simulink model "induct_closedloop_sim"  (Simulink 10.2)
settings: Solver=ode1  StartTime=0.0  StopTime=4  FixedStep=.000001  RelTol=1e-6  AbsTol=1e-6  EnableMultiTasking=on
values from neighbouring files (symbols this model uses):
  beta = M/(sigma*Lr*Ls)    (= 197.93605143)    [data_induct_closedloop.m]    (also in data_induct_closedloop_180turn.m)
  c1 = 3*wmax/(t1*t1)    (= 1066.66666667)    [data_induct_closedloop.m]    (also in data_induct_closedloop_180turn.m = 360000)
  c2 = -2*wmax/(t1*t1*t1)    (= -474.074074074)    [data_induct_closedloop.m]    (also in data_induct_closedloop_180turn.m = -9600000)
  d1 = 3*wmax/((t3-t2)*(t3-t2))    (= 1066.66666667)    [data_induct_closedloop.m]    (also in data_induct_closedloop_180turn.m = 360000)
  d2 = -2*wmax/((t3-t2)*(t3-t2)*(t3-t2))    (= -474.074074074)    [data_induct_closedloop.m]    (also in data_induct_closedloop_180turn.m = -9600000)
  eta = Rr/Lr    (= 278.571428571)    [data_induct_closedloop.m]    (also in data_induct_closedloop_180turn.m)
  eta2 = Rr/Lr    (= 278.571428571)    [data_induct_closedloop.m]    (also in data_induct_closedloop_180turn.m)
  f = 0    [data_induct_closedloop.m]    (also in data_induct_closedloop_180turn.m)
  gamma = M*M*Rr/(sigma*Lr*Lr*Ls) + Rs/(sigma*Ls)    (= 1047.76929212)    [data_induct_closedloop.m]    (also in data_induct_closedloop_180turn.m)
  id0 = 5.5/sqrt(2)    [data_induct_closedloop.m]    (also in data_induct_closedloop_180turn.m)
  Imax = 6    [data_induct_closedloop.m]    (also in data_induct_closedloop_180turn.m)
  J = 0.00011    [data_induct_closedloop.m]    (also in data_induct_closedloop_180turn.m)
  k0 = p0*p1*p2    (= 1000)    [data_induct_closedloop.m]    (also in data_induct_closedloop_180turn.m = 1000000)
  k1 = p0*p1 + p0*p2 + p1*p2    (= 300)    [data_induct_closedloop.m]    (also in data_induct_closedloop_180turn.m = 30000)
  k2 = p0+p1+p2    (= 30)    [data_induct_closedloop.m]    (also in data_induct_closedloop_180turn.m = 300)
  KI = 100*100    (= 10000)    [data_induct_closedloop.m]    (also in data_induct_closedloop_180turn.m = 1000000)
  KIf = 420000    [data_induct_closedloop.m]    (also in data_induct_closedloop_180turn.m)
  Kp = 100+100    (= 200)    [data_induct_closedloop.m]    (also in data_induct_closedloop_180turn.m = 2000)
  KPf = 10000    [data_induct_closedloop.m]    (also in data_induct_closedloop_180turn.m)
  KT2 = np*M2/Lr2    (= 2.50714285714)    [data_induct_closedloop.m]    (also in data_induct_closedloop_180turn.m)
  Lr = 0.014    [data_induct_closedloop.m]    (also in data_induct_closedloop_180turn.m)
  Ls = 0.014    [data_induct_closedloop.m]    (also in data_induct_closedloop_180turn.m)
  M = 0.0117    [data_induct_closedloop.m]    (also in data_induct_closedloop_180turn.m)
  M2 = M    (= 0.0117)    [data_induct_closedloop.m]    (also in data_induct_closedloop_180turn.m)
  mu = np*M/(J*Lr)    (= 22792.2077922)    [data_induct_closedloop.m]    (also in data_induct_closedloop_180turn.m)
  np = 3    [data_induct_closedloop.m]    (also in data_induct_closedloop_180turn.m)
  sigma = 1 - M*M/(Lr*Ls)    (= 0.301581632653)    [data_induct_closedloop.m]    (also in data_induct_closedloop_180turn.m)
  t3 = t2 + t1    (= 3.1)    [data_induct_closedloop.m]    (also in data_induct_closedloop_180turn.m = 0.0668879020479)
  tau_L = 0    [data_induct_closedloop.m]    (also in data_induct_closedloop_180turn.m)
  tdd = 0.01    [data_induct_closedloop.m]    (also in data_induct_closedloop_180turn.m)
  Vmax = V    (= 60)    [data_induct_closedloop.m]    (also in data_induct_closedloop_180turn.m)
  wbase = 250    [data_induct_closedloop.m]    (also in data_induct_closedloop_180turn.m)
undefined symbols (not defined in the file or in its folder): integrator_sat
libraries: simulink x2
settings Model: Creator=johnchiasson  LastModifiedBy=johnchiasson  ExtModeTrigMode=oneshot  ExtModeArmWhenConnect=off
settings DataIOCC: SignalLoggingName=sigsOut
settings OptimizationCC: BlockReduction=off  BooleanDataType=off  LifeSpan=auto
settings DebuggingCC: SaveWithParameterizedLinksMsg=none  SignalResolutionControl=TryResolveAllWithWarning  MultiTaskDSMMsg=warning  MultiTaskCondExecSysMsg=none  FcnCallInpInsideContextMsg=error  SFUnexpectedBacktrackingDiag=error  SFNoUnconditionalDefaultTransitionDiag=error  SFExecutionAtInitializationDiag=warning  ArithmeticOperatorsInVariantConditions=error
settings HardwareCC: TargetUnknown=on
settings SFSimCC: SimUseLocalCustomCode=on  CustomCodeUndefinedFunction=FilterOut
settings RTWCC: RTWUseLocalCustomCode=on
settings CodeAppCC: StateflowObjectComments=off
settings GRTTargetCC: TargetLangStandard=C99 (ISO)
settings ConfigComp: CovExternalEMLEnable=on

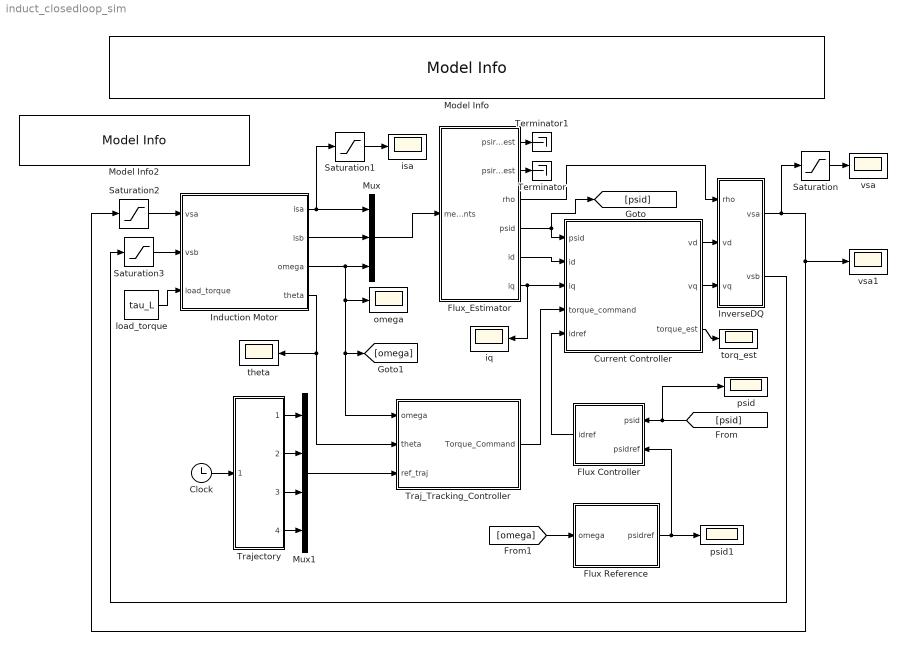
== system induct_closedloop_sim ==
  Clock : Clock
  Current Controller : Subsystem
  Flux Controller : Subsystem
  Flux Reference : Subsystem
  Flux_Estimator : Subsystem
  Induction Motor : Subsystem
  InverseDQ : Subsystem
  Model Info : simulink/Model-Wide Utilities/Model Info  Frame=on  DisplayStringWithTags=Simulation of an Input-Output Linearization Controller High Speed Run  HorizontalTextAlignment=Center  LeftAlignmentValue=0.5
  Model Info2 : simulink/Model-Wide Utilities/Model Info  Frame=on  DisplayStringWithTags="To initialize the simulation run  data_induct_closedloop.m"  HorizontalTextAlignment=Center  LeftAlignmentValue=0.5
  Mux : Mux  Inputs=3
  Mux1 : Mux
  Saturation : Saturate  UpperLimit=Vmax  LowerLimit=-Vmax
  Saturation1 : Saturate  UpperLimit=Imax  LowerLimit=-Imax
  Saturation2 : Saturate  UpperLimit=Vmax  LowerLimit=-Vmax
  Saturation3 : Saturate  UpperLimit=Vmax  LowerLimit=-Vmax
  Terminator : Terminator
  Terminator1 : Terminator
  Traj_Tracking_Controller : Subsystem
  Trajectory : Subsystem
  iq : Scope
  isa : Scope
  load_torque : Constant  Value=tau_L
  omega : Scope
  psid : Scope
  psid1 : Scope
  theta : Scope
  torq_est : Scope
  vsa : Scope
  vsa1 : Scope
  wires:
  load_torque/1 -> Induction Motor/3(load_torque)
  Mux/1 -> Flux_Estimator/1(measurements)
  Induction Motor/3(omega) -> Mux/3, Traj_Tracking_Controller/1(omega), [omega], omega/1
  Induction Motor/2(isb) -> Mux/2
  Induction Motor/1(isa) -> Mux/1, Saturation1/1
  Flux_Estimator/5(id) -> Current Controller/2(id)
  Flux_Estimator/6(iq) -> Current Controller/3(iq), iq/1
  Flux_Estimator/4(psid) -> Current Controller/1(psid), [psid]
  Current Controller/3(torque_est) -> torq_est/1
  Flux_Estimator/3(rho) -> InverseDQ/1(rho)
  Current Controller/1(vd) -> InverseDQ/2(vd)
  Current Controller/2(vq) -> InverseDQ/3(vq)
  Clock/1 -> Trajectory/1(time)
  Mux1/1 -> Traj_Tracking_Controller/3(ref_traj)
  Trajectory/4(jerk_ref) -> Mux1/4
  Trajectory/1(theta_ref) -> Mux1/1
  Trajectory/2(omega_ref) -> Mux1/2
  Trajectory/3(alpha_ref) -> Mux1/3
  InverseDQ/1(vsa) -> Saturation/1, Saturation2/1, vsa1/1
  InverseDQ/2(vsb) -> Saturation3/1
  Induction Motor/4(theta) -> Traj_Tracking_Controller/2(theta), theta/1
  Traj_Tracking_Controller/1(Torque_Command) -> Current Controller/4(torque_command)
  [psid] -> Flux Controller/1(psid), psid/1
  Flux Controller/1(idref) -> Current Controller/5(idref)
  Flux_Estimator/1(psira_est) -> Terminator1/1
  Flux_Estimator/2(psirb_est) -> Terminator/1
  Flux Reference/1(psidref) -> psid1/1, Flux Controller/2(psidref)
  [omega] -> Flux Reference/1(omega)
  Saturation/1 -> vsa/1
  Saturation1/1 -> isa/1
  Saturation2/1 -> Induction Motor/1(vsa)
  Saturation3/1 -> Induction Motor/2(vsb)

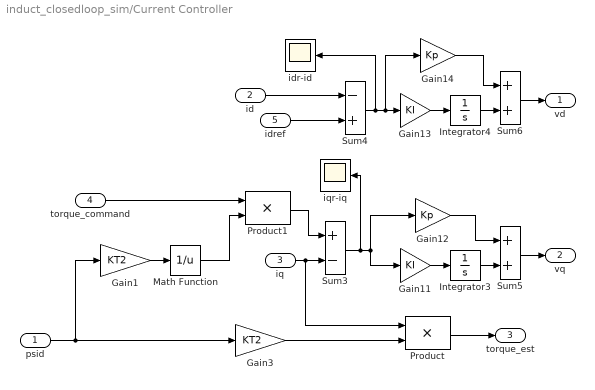
== system induct_closedloop_sim/Current Controller ==
  psid : Inport
  id : Inport  Port=2
  iq : Inport  Port=3
  torque_command : Inport  Port=4
  idref : Inport  Port=5
  Gain1 : Gain  Gain=KT2  SaturateOnIntegerOverflow=on  OutDataTypeStr=Inherit: Same as input  ParamDataTypeStr=Inherit: Same as input
  Gain11 : Gain  Gain=KI  SaturateOnIntegerOverflow=on  OutDataTypeStr=Inherit: Same as input  ParamDataTypeStr=Inherit: Same as input
  Gain12 : Gain  Gain=Kp  SaturateOnIntegerOverflow=on  OutDataTypeStr=Inherit: Same as input  ParamDataTypeStr=Inherit: Same as input
  Gain13 : Gain  Gain=KI  SaturateOnIntegerOverflow=on  OutDataTypeStr=Inherit: Same as input  ParamDataTypeStr=Inherit: Same as input
  Gain14 : Gain  Gain=Kp  SaturateOnIntegerOverflow=on  OutDataTypeStr=Inherit: Same as input  ParamDataTypeStr=Inherit: Same as input
  Gain3 : Gain  Gain=KT2  SaturateOnIntegerOverflow=on  OutDataTypeStr=Inherit: Same as input  ParamDataTypeStr=Inherit: Same as input
  Integrator3 : Integrator
  Integrator4 : Integrator
  Math Function : Math  Operator=reciprocal  SignedPower=on  SaturateOnIntegerOverflow=on
  Product : Product  InputSameDT=on  SaturateOnIntegerOverflow=on  OutDataTypeStr=Inherit: Same as first input
  Product1 : Product  InputSameDT=on  SaturateOnIntegerOverflow=on  OutDataTypeStr=Inherit: Same as first input
  Sum3 : Sum  Inputs=+-  InputSameDT=on  SaturateOnIntegerOverflow=on  OutDataTypeStr=Inherit: Same as first input
  Sum4 : Sum  Inputs=-+  InputSameDT=on  SaturateOnIntegerOverflow=on  OutDataTypeStr=Inherit: Same as first input
  Sum5 : Sum  InputSameDT=on  SaturateOnIntegerOverflow=on  OutDataTypeStr=Inherit: Same as first input
  Sum6 : Sum  InputSameDT=on  SaturateOnIntegerOverflow=on  OutDataTypeStr=Inherit: Same as first input
  idr-id : Scope
  iqr-iq : Scope
  vd : Outport
  vq : Outport  Port=2
  torque_est : Outport  Port=3
  wires:
  Sum4/1 -> idr-id/1, Gain13/1, Gain14/1
  Sum3/1 -> iqr-iq/1, Gain11/1, Gain12/1
  Gain12/1 -> Sum5/1
  Integrator3/1 -> Sum5/2
  Gain11/1 -> Integrator3/1
  Gain14/1 -> Sum6/1
  Gain13/1 -> Integrator4/1
  Sum6/1 -> vd/1
  id/1 -> Sum4/1
  idref/1 -> Sum4/2
  Product1/1 -> Sum3/1
  Sum5/1 -> vq/1
  iq/1 -> Sum3/2, Product/1
  Integrator4/1 -> Sum6/2
  Gain3/1 -> Product/2
  Product/1 -> torque_est/1
  psid/1 -> Gain3/1, Gain1/1
  torque_command/1 -> Product1/1
  Math Function/1 -> Product1/2
  Gain1/1 -> Math Function/1

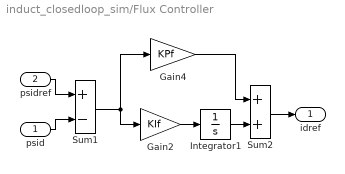
== system induct_closedloop_sim/Flux Controller ==
  psid : Inport
  psidref : Inport  Port=2
  Gain2 : Gain  Gain=KIf  SaturateOnIntegerOverflow=on  OutDataTypeStr=Inherit: Same as input  ParamDataTypeStr=Inherit: Same as input
  Gain4 : Gain  Gain=KPf  SaturateOnIntegerOverflow=on  OutDataTypeStr=Inherit: Same as input  ParamDataTypeStr=Inherit: Same as input
  Integrator1 : Integrator
  Sum1 : Sum  Inputs=+-  InputSameDT=on  SaturateOnIntegerOverflow=on  OutDataTypeStr=Inherit: Same as first input
  Sum2 : Sum  InputSameDT=on  SaturateOnIntegerOverflow=on  OutDataTypeStr=Inherit: Same as first input
  idref : Outport
  wires:
  Sum1/1 -> Gain2/1, Gain4/1
  Gain4/1 -> Sum2/1
  Integrator1/1 -> Sum2/2
  Gain2/1 -> Integrator1/1
  Sum2/1 -> idref/1
  psidref/1 -> Sum1/1
  psid/1 -> Sum1/2

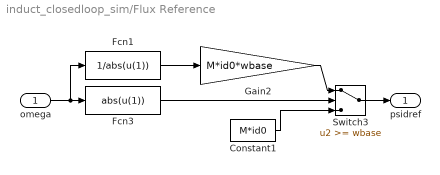
== system induct_closedloop_sim/Flux Reference ==
  omega : Inport
  Constant1 : Constant  Value=M*id0
  Fcn1 : Fcn  Expr=1/abs(u(1))
  Fcn3 : Fcn  Expr=abs(u(1))
  Gain2 : Gain  Gain=M*id0*wbase  SaturateOnIntegerOverflow=on  OutDataTypeStr=Inherit: Same as input  ParamDataTypeStr=Inherit: Same as input
  Switch3 : Switch  Threshold=wbase  SaturateOnIntegerOverflow=on  InputSameDT=on
  psidref : Outport
  wires:
  Gain2/1 -> Switch3/1
  Fcn3/1 -> Switch3/2
  omega/1 -> Fcn1/1, Fcn3/1
  Fcn1/1 -> Gain2/1
  Constant1/1 -> Switch3/3
  Switch3/1 -> psidref/1

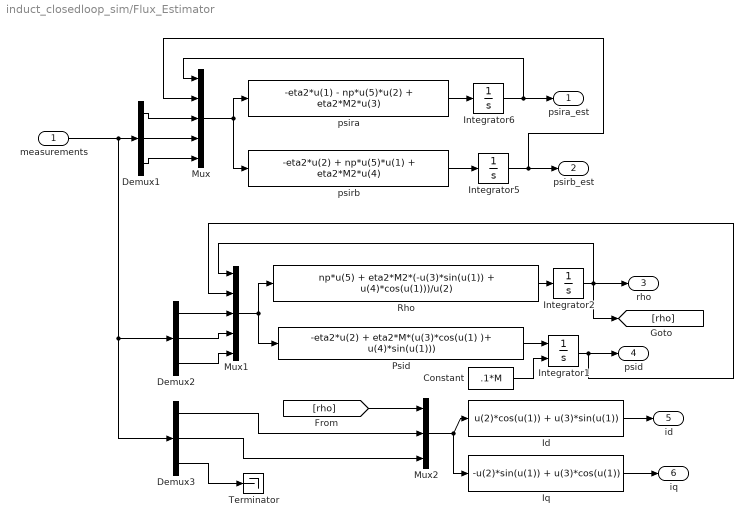
== system induct_closedloop_sim/Flux_Estimator ==
  measurements : Inport
  Constant : Constant  Value=.1*M
  Demux1 : Demux  Outputs=3
      settings: DisplayOption=none
  Demux2 : Demux  Outputs=3
      settings: DisplayOption=none
  Demux3 : Demux  Outputs=3
      settings: DisplayOption=none
  Id : Fcn  Expr=u(2)*cos(u(1)) + u(3)*sin(u(1))
  Integrator1 : Integrator  InitialConditionSource=external  UpperSaturationLimit=integrator_sat  LowerSaturationLimit=-integrator_sat
  Integrator2 : Integrator  UpperSaturationLimit=integrator_sat  LowerSaturationLimit=-integrator_sat
  Integrator5 : Integrator  UpperSaturationLimit=integrator_sat  LowerSaturationLimit=-integrator_sat
  Integrator6 : Integrator  UpperSaturationLimit=integrator_sat  LowerSaturationLimit=-integrator_sat
  Iq : Fcn  Expr=-u(2)*sin(u(1)) + u(3)*cos(u(1))
  Mux : Mux  Inputs=5
  Mux1 : Mux  Inputs=5
  Mux2 : Mux  Inputs=3
  Psid : Fcn  Expr=-eta2*u(2) + eta2*M*(u(3)*cos(u(1) )+ u(4)*sin(u(1)))
  Rho : Fcn  Expr=np*u(5) + eta2*M2*(-u(3)*sin(u(1)) + u(4)*cos(u(1)))/u(2)
  Terminator : Terminator
  psira : Fcn  Expr=-eta2*u(1) - np*u(5)*u(2) + eta2*M2*u(3)
  psirb : Fcn  Expr=-eta2*u(2) + np*u(5)*u(1) + eta2*M2*u(4)
  psira_est : Outport
  psirb_est : Outport  Port=2
  rho : Outport  Port=3
  psid : Outport  Port=4
  id : Outport  Port=5
  iq : Outport  Port=6
  wires:
  psirb/1 -> Integrator5/1
  psira/1 -> Integrator6/1
  Integrator6/1 -> psira_est/1, Mux/1
  Integrator5/1 -> psirb_est/1, Mux/2
  Mux/1 -> psira/1, psirb/1
  Psid/1 -> Integrator1/1
  Rho/1 -> Integrator2/1
  Integrator2/1 -> rho/1, Mux1/1, [rho]
  Integrator1/1 -> psid/1, Mux1/2
  Mux1/1 -> Rho/1, Psid/1
  Id/1 -> id/1
  Iq/1 -> iq/1
  Demux3/1 -> Mux2/2
  Demux3/3 -> Terminator/1
  Demux3/2 -> Mux2/3
  [rho] -> Mux2/1
  Mux2/1 -> Id/1, Iq/1
  Constant/1 -> Integrator1/2
  measurements/1 -> Demux1/1, Demux2/1, Demux3/1
  Demux1/1 -> Mux/3
  Demux1/2 -> Mux/4
  Demux1/3 -> Mux/5
  Demux2/1 -> Mux1/3
  Demux2/2 -> Mux1/4
  Demux2/3 -> Mux1/5

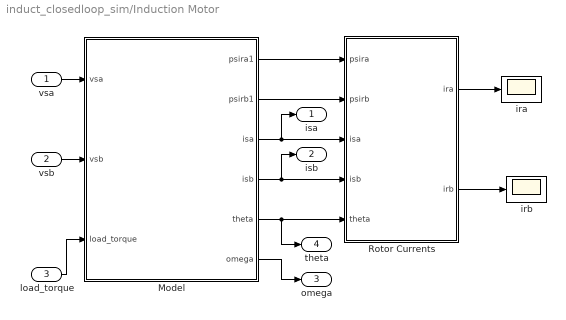
== system induct_closedloop_sim/Induction Motor ==
  vsa : Inport
  vsb : Inport  Port=2
  load_torque : Inport  Port=3
  Model : Subsystem
  Rotor Currents : Subsystem
  ira : Scope
  irb : Scope
  isa : Outport
  isb : Outport  Port=2
  omega : Outport  Port=3
  theta : Outport  Port=4
  wires:
  Model/1(psira1) -> Rotor Currents/1(psira)
  Model/2(psirb1) -> Rotor Currents/2(psirb)
  Model/3(isa) -> Rotor Currents/3(isa), isa/1
  Model/4(isb) -> Rotor Currents/4(isb), isb/1
  Model/6(omega) -> omega/1
  vsa/1 -> Model/1(vsa)
  vsb/1 -> Model/2(vsb)
  load_torque/1 -> Model/3(load_torque)
  Model/5(theta) -> theta/1, Rotor Currents/5(theta)
  Rotor Currents/1(ira) -> ira/1
  Rotor Currents/2(irb) -> irb/1

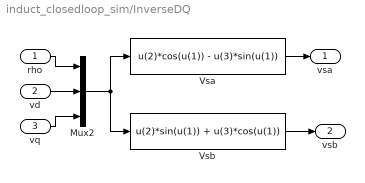
== system induct_closedloop_sim/InverseDQ ==
  rho : Inport
  vd : Inport  Port=2
  vq : Inport  Port=3
  Mux2 : Mux  Inputs=3
  Vsa : Fcn  Expr=u(2)*cos(u(1)) - u(3)*sin(u(1))
  Vsb : Fcn  Expr=u(2)*sin(u(1)) + u(3)*cos(u(1))
  vsa : Outport
  vsb : Outport  Port=2
  wires:
  Vsa/1 -> vsa/1
  Vsb/1 -> vsb/1
  Mux2/1 -> Vsa/1, Vsb/1
  rho/1 -> Mux2/1
  vd/1 -> Mux2/2
  vq/1 -> Mux2/3

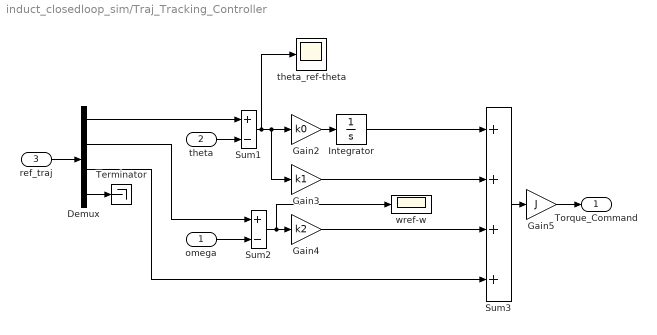
== system induct_closedloop_sim/Traj_Tracking_Controller ==
  omega : Inport
  theta : Inport  Port=2
  ref_traj : Inport  Port=3
  Demux : Demux
      settings: DisplayOption=none
  Gain2 : Gain  Gain=k0  SaturateOnIntegerOverflow=on  OutDataTypeStr=Inherit: Same as input  ParamDataTypeStr=Inherit: Same as input
  Gain3 : Gain  Gain=k1  SaturateOnIntegerOverflow=on  OutDataTypeStr=Inherit: Same as input  ParamDataTypeStr=Inherit: Same as input
  Gain4 : Gain  Gain=k2  SaturateOnIntegerOverflow=on  OutDataTypeStr=Inherit: Same as input  ParamDataTypeStr=Inherit: Same as input
  Gain5 : Gain  Gain=J  SaturateOnIntegerOverflow=on  OutDataTypeStr=Inherit: Same as input  ParamDataTypeStr=Inherit: Same as input
  Integrator : Integrator
  Sum1 : Sum  Inputs=+-  InputSameDT=on  SaturateOnIntegerOverflow=on  OutDataTypeStr=Inherit: Same as first input
  Sum2 : Sum  Inputs=+-  InputSameDT=on  SaturateOnIntegerOverflow=on  OutDataTypeStr=Inherit: Same as first input
  Sum3 : Sum  Inputs=++++  InputSameDT=on  SaturateOnIntegerOverflow=on  OutDataTypeStr=Inherit: Same as first input
  Terminator : Terminator
  theta_ref-theta : Scope
  wref-w : Scope
  Torque_Command : Outport
  wires:
  Demux/1 -> Sum1/1
  Gain2/1 -> Integrator/1
  Integrator/1 -> Sum3/1
  theta/1 -> Sum1/2
  ref_traj/1 -> Demux/1
  Demux/4 -> Terminator/1
  Demux/2 -> Sum2/1
  Gain4/1 -> Sum3/3
  Sum3/1 -> Gain5/1
  Sum1/1 -> Gain2/1, Gain3/1, theta_ref-theta/1
  Sum2/1 -> Gain4/1, wref-w/1
  Gain3/1 -> Sum3/2
  Gain5/1 -> Torque_Command/1
  omega/1 -> Sum2/2
  Demux/3 -> Sum3/4

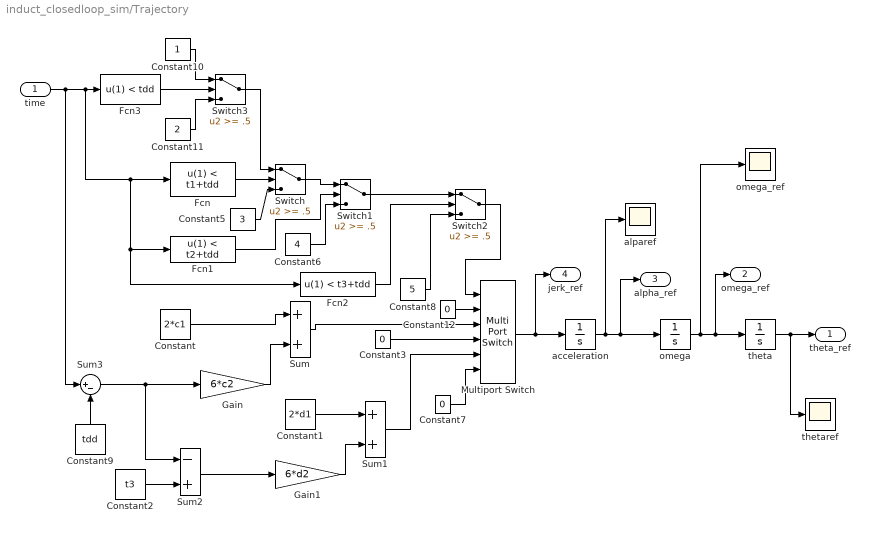
== system induct_closedloop_sim/Trajectory ==
  time : Inport
  Constant : Constant  Value=2*c1
  Constant1 : Constant  Value=2*d1
  Constant10 : Constant
  Constant11 : Constant  Value=2
  Constant12 : Constant  Value=0
  Constant2 : Constant  Value=t3
  Constant3 : Constant  Value=0
  Constant5 : Constant  Value=3
  Constant6 : Constant  Value=4
  Constant7 : Constant  Value=0
  Constant8 : Constant  Value=5
  Constant9 : Constant  Value=tdd
  Fcn : Fcn  Expr=u(1) < t1+tdd
  Fcn1 : Fcn  Expr=u(1) < t2+tdd
  Fcn2 : Fcn  Expr=u(1) < t3+tdd
  Fcn3 : Fcn  Expr=u(1) < tdd
  Gain : Gain  Gain=6*c2  SaturateOnIntegerOverflow=on  OutDataTypeStr=Inherit: Same as input  ParamDataTypeStr=Inherit: Same as input
  Gain1 : Gain  Gain=6*d2  SaturateOnIntegerOverflow=on  OutDataTypeStr=Inherit: Same as input  ParamDataTypeStr=Inherit: Same as input
  Multiport Switch : MultiPortSwitch  Inputs=5  SaturateOnIntegerOverflow=on  InputSameDT=on
  Sum : Sum  Inputs=|++  InputSameDT=on  SaturateOnIntegerOverflow=on  OutDataTypeStr=Inherit: Same as first input
  Sum1 : Sum  Inputs=|++  InputSameDT=on  SaturateOnIntegerOverflow=on  OutDataTypeStr=Inherit: Same as first input
  Sum2 : Sum  Inputs=-+  InputSameDT=on  SaturateOnIntegerOverflow=on  OutDataTypeStr=Inherit: Same as first input
  Sum3 : Sum  Inputs=|+-  InputSameDT=on  SaturateOnIntegerOverflow=on  OutDataTypeStr=Inherit: Same as first input
  Switch{,1..3} (4 alike) : Switch  Threshold=.5  SaturateOnIntegerOverflow=on  InputSameDT=on
  acceleration : Integrator
  alparef : Scope
  omega : Integrator
  "omega_ref " : Scope
  theta : Integrator
  thetaref : Scope
  theta_ref : Outport
  omega_ref : Outport  Port=2
  alpha_ref : Outport  Port=3
  jerk_ref : Outport  Port=4
  wires:
  Constant/1 -> Sum/1
  Gain/1 -> Sum/2
  Constant2/1 -> Sum2/2
  Sum2/1 -> Gain1/1
  Constant1/1 -> Sum1/1
  Gain1/1 -> Sum1/2
  Fcn/1 -> Switch/2
  Constant5/1 -> Switch/3
  Constant6/1 -> Switch1/3
  Fcn1/1 -> Switch1/2
  Switch/1 -> Switch1/1
  Sum1/1 -> Multiport Switch/5
  Sum/1 -> Multiport Switch/3
  Constant3/1 -> Multiport Switch/4
  omega/1 -> theta/1, omega_ref/1, "omega_ref "/1
  Multiport Switch/1 -> acceleration/1, jerk_ref/1
  acceleration/1 -> omega/1, alpha_ref/1, alparef/1
  theta/1 -> theta_ref/1, thetaref/1
  Constant7/1 -> Multiport Switch/6
  Fcn2/1 -> Switch2/2
  Constant8/1 -> Switch2/3
  Switch1/1 -> Switch2/1
  Switch2/1 -> Multiport Switch/1
  Constant12/1 -> Multiport Switch/2
  Switch3/1 -> Switch/1
  Constant10/1 -> Switch3/1
  Constant11/1 -> Switch3/3
  Fcn3/1 -> Switch3/2
  Constant9/1 -> Sum3/2
  Sum3/1 -> Gain/1, Sum2/1
  time/1 -> Fcn3/1, Fcn/1, Fcn1/1, Fcn2/1, Sum3/1

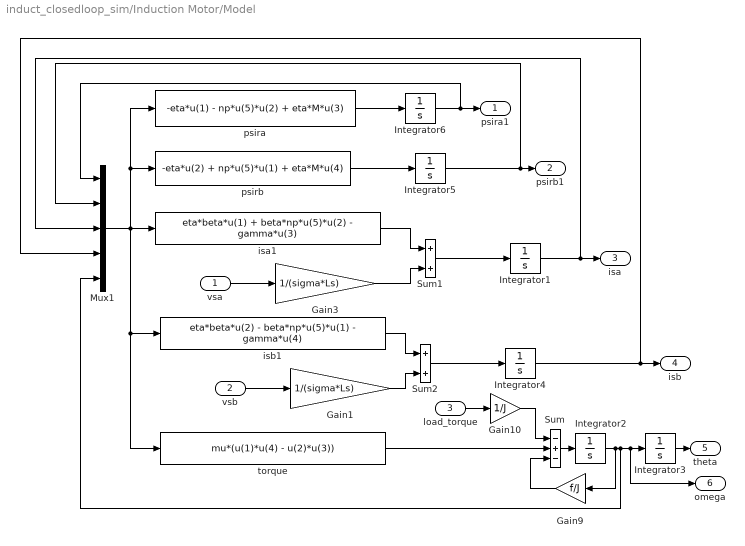
== system induct_closedloop_sim/Induction Motor/Model ==
  vsa : Inport
  vsb : Inport  Port=2
  load_torque : Inport  Port=3
  Gain1 : Gain  Gain=1/(sigma*Ls)  SaturateOnIntegerOverflow=on  OutDataTypeStr=Inherit: Same as input  ParamDataTypeStr=Inherit: Same as input
  Gain10 : Gain  Gain=1/J  SaturateOnIntegerOverflow=on  OutDataTypeStr=Inherit: Same as input  ParamDataTypeStr=Inherit: Same as input
  Gain3 : Gain  Gain=1/(sigma*Ls)  SaturateOnIntegerOverflow=on  OutDataTypeStr=Inherit: Same as input  ParamDataTypeStr=Inherit: Same as input
  Gain9 : Gain  Gain=f/J  SaturateOnIntegerOverflow=on  OutDataTypeStr=Inherit: Same as input  ParamDataTypeStr=Inherit: Same as input
  Integrator{1..4} (4 alike) : Integrator
  Integrator5 : Integrator  UpperSaturationLimit=integrator_sat  LowerSaturationLimit=-integrator_sat
  Integrator6 : Integrator  UpperSaturationLimit=integrator_sat  LowerSaturationLimit=-integrator_sat
  Mux1 : Mux  Inputs=5
  Sum : Sum  Inputs=-+-  InputSameDT=on  SaturateOnIntegerOverflow=on  OutDataTypeStr=Inherit: Same as first input
  Sum1 : Sum  InputSameDT=on  SaturateOnIntegerOverflow=on  OutDataTypeStr=Inherit: Same as first input
  Sum2 : Sum  InputSameDT=on  SaturateOnIntegerOverflow=on  OutDataTypeStr=Inherit: Same as first input
  isa1 : Fcn  Expr=eta*beta*u(1) + beta*np*u(5)*u(2) - gamma*u(3)
  isb1 : Fcn  Expr=eta*beta*u(2) - beta*np*u(5)*u(1) - gamma*u(4)
  psira : Fcn  Expr=-eta*u(1) - np*u(5)*u(2) + eta*M*u(3)
  psirb : Fcn  Expr=-eta*u(2) + np*u(5)*u(1) + eta*M*u(4)
  torque : Fcn  Expr=mu*(u(1)*u(4) - u(2)*u(3))
  psira1 : Outport
  psirb1 : Outport  Port=2
  isa : Outport  Port=3
  isb : Outport  Port=4
  theta : Outport  Port=5
  omega : Outport  Port=6
  wires:
  vsa/1 -> Gain3/1
  vsb/1 -> Gain1/1
  Mux1/1 -> isa1/1, psirb/1, psira/1, isb1/1, torque/1
  Sum/1 -> Integrator2/1
  Integrator2/1 -> Gain9/1, Integrator3/1, omega/1, Mux1/5
  Integrator3/1 -> theta/1
  load_torque/1 -> Gain10/1
  Gain10/1 -> Sum/1
  Gain9/1 -> Sum/3
  torque/1 -> Sum/2
  Sum2/1 -> Integrator4/1
  Gain1/1 -> Sum2/2
  isb1/1 -> Sum2/1
  Integrator4/1 -> isb/1, Mux1/4
  Sum1/1 -> Integrator1/1
  Integrator1/1 -> Mux1/3, isa/1
  Gain3/1 -> Sum1/2
  isa1/1 -> Sum1/1
  psirb/1 -> Integrator5/1
  Integrator5/1 -> Mux1/2, psirb1/1
  Integrator6/1 -> psira1/1, Mux1/1
  psira/1 -> Integrator6/1

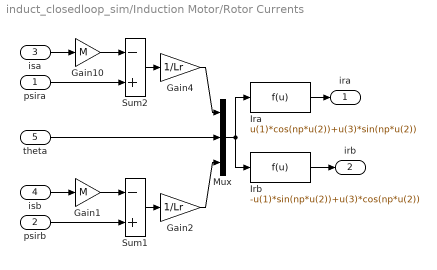
== system induct_closedloop_sim/Induction Motor/Rotor Currents ==
  psira : Inport
  psirb : Inport  Port=2
  isa : Inport  Port=3
  isb : Inport  Port=4
  theta : Inport  Port=5
  Gain1 : Gain  Gain=M  SaturateOnIntegerOverflow=on  OutDataTypeStr=Inherit: Same as input  ParamDataTypeStr=Inherit: Same as input
  Gain10 : Gain  Gain=M  SaturateOnIntegerOverflow=on  OutDataTypeStr=Inherit: Same as input  ParamDataTypeStr=Inherit: Same as input
  Gain2 : Gain  Gain=1/Lr  SaturateOnIntegerOverflow=on  OutDataTypeStr=Inherit: Same as input  ParamDataTypeStr=Inherit: Same as input
  Gain4 : Gain  Gain=1/Lr  SaturateOnIntegerOverflow=on  OutDataTypeStr=Inherit: Same as input  ParamDataTypeStr=Inherit: Same as input
  Ira : Fcn  Expr=u(1)*cos(np*u(2))+u(3)*sin(np*u(2))
  Irb : Fcn  Expr=-u(1)*sin(np*u(2))+u(3)*cos(np*u(2))
  Mux : Mux  Inputs=3
  Sum1 : Sum  Inputs=-+  InputSameDT=on  SaturateOnIntegerOverflow=on  OutDataTypeStr=Inherit: Same as first input
  Sum2 : Sum  Inputs=-+  InputSameDT=on  SaturateOnIntegerOverflow=on  OutDataTypeStr=Inherit: Same as first input
  ira : Outport
  irb : Outport  Port=2
  wires:
  Gain10/1 -> Sum2/1
  Sum2/1 -> Gain4/1
  Irb/1 -> irb/1
  Ira/1 -> ira/1
  Mux/1 -> Ira/1, Irb/1
  Gain4/1 -> Mux/1
  Gain1/1 -> Sum1/1
  Sum1/1 -> Gain2/1
  Gain2/1 -> Mux/3
  isa/1 -> Gain10/1
  psira/1 -> Sum2/2
  theta/1 -> Mux/2
  isb/1 -> Gain1/1
  psirb/1 -> Sum1/2
